simulink model "cartesian_impedance_control"  (R2019a)
settings: Solver=FixedStepDiscrete  StartTime=0.0  StopTime=inf  FixedStep=0.001  RelTol=1e-3  EnableMultiTasking=on
PreLoadFcn:
  | demos_common_configs();
  | 
  | collision_behavior = ones(1,52)*100;
libraries: franka_simulink_library x5, franka_simulink_library_misc x5, robotcorelib x1
settings Model: SimulationMode=external  ExtModeTrigDuration=10000  Creator=vasi_ko  LastModifiedBy=kvasios
settings DataIOCC: LimitDataPoints=on  SaveFormat=Array  ReturnWorkspaceOutputs=off
settings OptimizationCC: DefaultParameterBehavior=Inlined  EnhancedBackFolding=on  PassReuseOutputArgsAs=Individual arguments  ZeroExternalMemoryAtStartup=off  ZeroInternalMemoryAtStartup=off  OptimizeBlockOrder=speed  DifferentSizesBufferReuse=on  OptimizationCustomize=off
settings DebuggingCC: SolverPrmCheckMsg=warning  ParameterTunabilityLossMsg=error  SFUnexpectedBacktrackingDiag=warning  SFNoUnconditionalDefaultTransitionDiag=warning  SFExecutionAtInitializationDiag=none  ArithmeticOperatorsInVariantConditions=warning
settings HardwareCC: ProdBitPerLong=64  ProdHWDeviceType=Intel->x86-64 (Linux 64)
settings ModelReferenceCC: PropagateSignalLabelsOutOfModel=off
settings SFSimCC: SimUseLocalCustomCode=off  MATLABDynamicMemAlloc=off
settings RTWCC: SystemTargetFile=franka_emika_panda.tlc  GenCodeOnly=on  TemplateMakefile=ert_default_tmf  RTWVerbose=off  RTWUseLocalCustomCode=off  Toolchain=Franka Simulink | gmake (64-bit linux)  BuildConfiguration=Faster Runs  IncludeHyperlinkInReport=on  TargetLang=C++
settings CodeAppCC: ForceParamTrailComments=on  IgnoreCustomStorageClasses=off  OperatorAnnotations=on  SimulinkDataObjDesc=on  SFDataObjDesc=on  InsertBlockDesc=on
settings STFCustomTargetCC: TargetLangStandard=C99 (ISO)  MultiwordLength=256  GenerateSampleERTMain=on  ModelReferenceCompliant=off  CombineOutputUpdateFcns=on  ERTCustomFileBanners=on  SupportNonInlinedSFcns=off  RemoveResetFunc=on  MATLABClassNameForMDSCustomization=Simulink.SoftwareTarget.ERTCustomization  CPPClassGenCompliant=on  GRTInterface=off  UseToolchainInfoCompliant=on  SystemTargetFile=franka_emika_panda.tlc
settings ERTTargetCC: TargetLangStandard=C99 (ISO)  GenerateSampleERTMain=on  ModelReferenceCompliant=off  ParMdlRefBuildCompliant=off  CompOptLevelCompliant=off  ConcurrentExecutionCompliant=off  SupportContinuousTime=on  ModelStepFunctionPrototypeControlCompliant=off  ExtMode=on  ExtModeMexArgs='192.168.1.199' 0 17725  InlinedParameterPlacement=NonHierarchical  ERTCustomFileTemplate=franka_emika_panda_file_process.tlc
settings ConfigComp: CovMetricSettings=dw  CovSaveCumulativeToWorkspaceVar=on  CovSaveSingleToWorkspaceVar=on  CovExternalEMLEnable=off  CovSFcnEnable=off

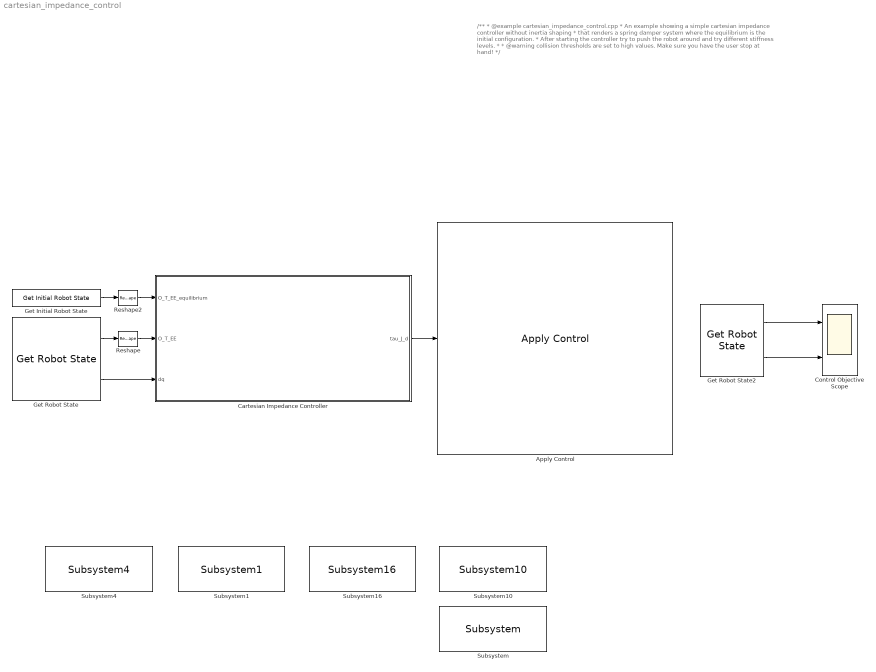
== system cartesian_impedance_control ==
  note: /**
      |  * @example cartesian_impedance_control.cpp
      |  * An example showing a simple cartesian impedance controller without inertia shaping
      |  * that renders a spring damper system where the equilibrium is the initial configuration.
      |  * After starting the controller try to push the robot around and try different stiffness levels.
      |  *
      |  * @warning collision thresholds are set to high values. Make sure you have the user stop at hand!
      |  */
  Apply Control : franka_simulink_library/Apply Control  robot_ip=robot_ip  gripper_attached=off  control_mode=Torque Control  controller_choice=Joint Impedance Controller  elbow_control=on  collision_thresholds=100*ones(1,52)  joint_impedance=joint_impedance  cartesian_impedance=cartesian_impedance  load_inertia=load_inertia  EE_T_K=EE_T_K  init_joint_configuration_req=on  init_joint_configuration=[0, -pi/4, 0, -3 * pi/4, 0, pi/2, pi/4]
      settings: SourceProductName=Franka Emika
  Cartesian Impedance Controller : Subsystem
      mask Display:
      | disp('{\bf\fontsize{18}Cartesian Impedance Controller}', 'texmode','on');
      | 
      | block_icon('Controller')
      | 
      | port_label('output',1,'tau_J_d');
      | 
      | port_label('input',1,'O_T_EE_equilibrium');
      | port_label('input',2,'O_T_EE');
      | port_label('input',3,'dq');
  Control Objective Scope : Scope  NumInputPorts=2
  Get Initial Robot State : franka_simulink_library/Get Initial Robot State  robot_ip=robot_ip  signals_requested='O_T_EE'
      settings: SourceProductName=Franka Emika
  Get Robot State : franka_simulink_library/Get Robot State  robot_ip=robot_ip  signals_requested='O_T_EE dq'
      settings: SourceProductName=Franka Emika
  Get Robot State2 : franka_simulink_library/Get Robot State  robot_ip=robot_ip  signals_requested='K_F_ext_hat_K O_T_EE'
      settings: SourceProductName=Franka Emika
  Reshape : Reshape  OutputDimensionality=Customize  OutputDimensions=[4,4]
  Reshape2 : Reshape  OutputDimensionality=Customize  OutputDimensions=[4,4]
  Subsystem : franka_simulink_library_misc/Subsystem  SystemSampleTime=-1  Latency=0  AutoFrameSizeCalculation=off
  Subsystem1 : franka_simulink_library_misc/Subsystem1  SystemSampleTime=-1  Latency=0  AutoFrameSizeCalculation=off
  Subsystem10 : franka_simulink_library_misc/Subsystem10  SystemSampleTime=-1  Latency=0  AutoFrameSizeCalculation=off
  Subsystem16 : franka_simulink_library_misc/Subsystem16  SystemSampleTime=-1  Latency=0  AutoFrameSizeCalculation=off
  Subsystem4 : franka_simulink_library_misc/Subsystem4  SystemSampleTime=-1  Latency=0  AutoFrameSizeCalculation=off
  wires:
  Cartesian Impedance Controller/1(tau_J_d) -> Apply Control/1
  Get Initial Robot State/1 -> Reshape2/1
  Get Robot State/1 -> Reshape/1
  Get Robot State/2 -> Cartesian Impedance Controller/3(dq)
  Reshape/1 -> Cartesian Impedance Controller/2(O_T_EE)
  Reshape2/1 -> Cartesian Impedance Controller/1(O_T_EE_equilibrium)
  Get Robot State2/1 -> Control Objective Scope/1
  Get Robot State2/2 -> Control Objective Scope/2

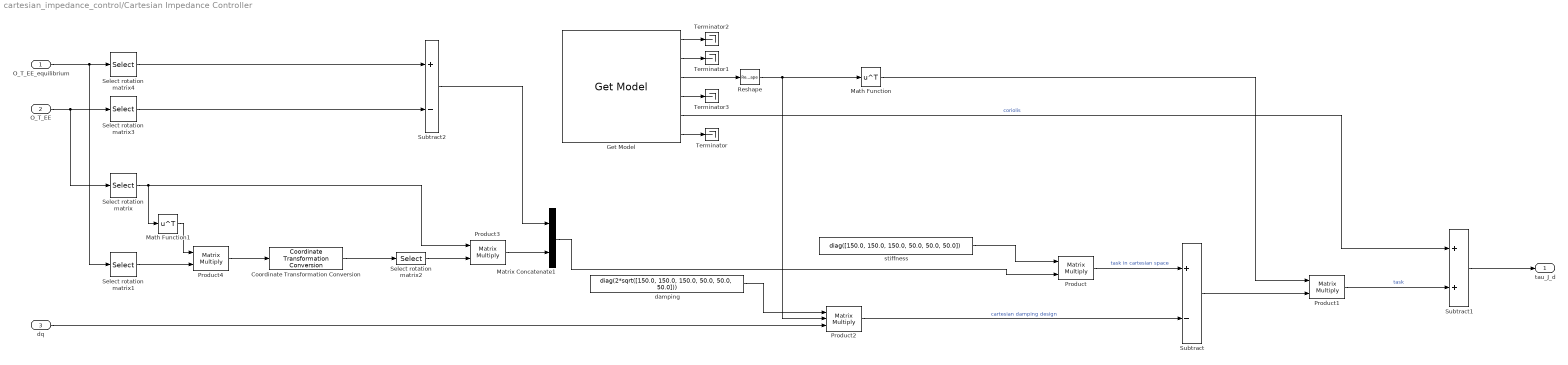
== system cartesian_impedance_control/Cartesian Impedance Controller ==
  O_T_EE_equilibrium : Inport
  O_T_EE : Inport  Port=2
  dq : Inport  Port=3
  Coordinate Transformation Conversion : robotcorelib/Coordinate Transformation Conversion  InputRepresentation=Rotation Matrix  InputEulerSequence=ZYX  ShowTrVecInputPort=on  OutputRepresentation=Quaternion  OutputEulerSequence=ZYX  ShowTrVecOutputPort=on  SimulateUsing=Code generation
      settings: SourceProductBaseCode=NV,RO,RR,UV
  Get Model : franka_simulink_library/Get Model  robot_ip=robot_ip
      settings: SourceProductName=Franka Emika
  Math Function : Math  Operator=transpose  SaturateOnIntegerOverflow=on
  Math Function1 : Math  Operator=transpose  SaturateOnIntegerOverflow=on
  Matrix Concatenate1 : Concatenate
  Product{,1,3..4} (4 alike) : Product  Multiplication=Matrix(*)
  Product2 : Product  Inputs=3  Multiplication=Matrix(*)
  Reshape : Reshape  OutputDimensionality=Customize  OutputDimensions=[6,7]
  Select rotation matrix : Selector  NumberOfDimensions=2  InputPortWidth=3  IndexOptions=Index vector (dialog),Index vector (dialog)  Indices=[1,2,3],[1 2 3]  OutputSizes=1
  Select rotation matrix1 : Selector  NumberOfDimensions=2  InputPortWidth=3  IndexOptions=Index vector (dialog),Index vector (dialog)  Indices=[1,2,3],[1 2 3]  OutputSizes=1
  Select rotation matrix2 : Selector  InputPortWidth=4  IndexOptions=Index vector (dialog)  Indices=[2,3,4]  OutputSizes=1
  Select rotation matrix3 : Selector  NumberOfDimensions=2  InputPortWidth=3  IndexOptions=Index vector (dialog),Index vector (dialog)  Indices=[1,2,3],[4]  OutputSizes=1
  Select rotation matrix4 : Selector  NumberOfDimensions=2  InputPortWidth=3  IndexOptions=Index vector (dialog),Index vector (dialog)  Indices=[1,2,3],[4]  OutputSizes=1
  Subtract : Sum  Inputs=+-
  Subtract1 : Sum
  Subtract2 : Sum  Inputs=+-
  Terminator{,1..3} (4 alike) : Terminator
  damping : Constant  Value=diag(2*sqrt([150.0, 150.0, 150.0, 50.0, 50.0, 50.0]))  VectorParams1D=off
  stiffness : Constant  Value=diag([150.0, 150.0, 150.0, 50.0, 50.0, 50.0])  VectorParams1D=off
  tau_J_d : Outport  VectorParamsAs1DForOutWhenUnconnected=off
  wires:
  Get Model/6 -> Terminator/1
  Get Model/2 -> Terminator1/1
  Get Model/1 -> Terminator2/1
  Get Model/4 -> Terminator3/1
  Get Model/3 -> Reshape/1
  Reshape/1 -> Product2/2, Math Function/1
  stiffness/1 -> Product/1
  Math Function/1 -> Product1/1
  Product/1 -> Subtract/1  "task in cartesian space"
  Product2/1 -> Subtract/2  "cartesian damping design"
  Get Model/5 -> Subtract1/1  "coriolis"
  dq/1 -> Product2/3
  damping/1 -> Product2/1
  Subtract1/1 -> tau_J_d/1
  Product1/1 -> Subtract1/2  "task"
  O_T_EE/1 -> Select rotation matrix3/1, Select rotation matrix/1
  O_T_EE_equilibrium/1 -> Select rotation matrix4/1, Select rotation matrix1/1
  Select rotation matrix4/1 -> Subtract2/1
  Select rotation matrix3/1 -> Subtract2/2
  Subtract2/1 -> Matrix Concatenate1/1
  Coordinate Transformation Conversion/1 -> Select rotation matrix2/1
  Product4/1 -> Coordinate Transformation Conversion/1
  Subtract/1 -> Product1/2
  Select rotation matrix2/1 -> Product3/2
  Matrix Concatenate1/1 -> Product/2
  Select rotation matrix/1 -> Math Function1/1, Product3/1
  Product3/1 -> Matrix Concatenate1/2
  Select rotation matrix1/1 -> Product4/2
  Math Function1/1 -> Product4/1
